simulink model "linear_sim"  (R2024b)
settings: Solver=VariableStepAuto  StartTime=0.0  StopTime=10.0  MaxStep=1e-4  RelTol=1e-3
values from neighbouring files (symbols this model uses):
  c_l_d = 1.5    [linear_params.m]
  K = -lqr(sys,Q,R,0)    [linear_model.m]
  K_pre = 1/dcgain(sys_cl(1,1))    [linear_model.m]
  ref_area = 0.005    [linear_params.m]
  ref_length = 0.25    [linear_params.m]
  rho = 1.293    [linear_params.m]
  tau = 1/60    (= 0.0166666666667)    [linear_params.m]
  V = 100    [linear_model.m]    (also in linear_params.m = 1000)
undefined symbols (not defined in the file or in its folder): backlash, gaussian
libraries: simulink x4, aerolibactuator x1
settings Model: Creator=finnb  LastModifiedBy=finnb

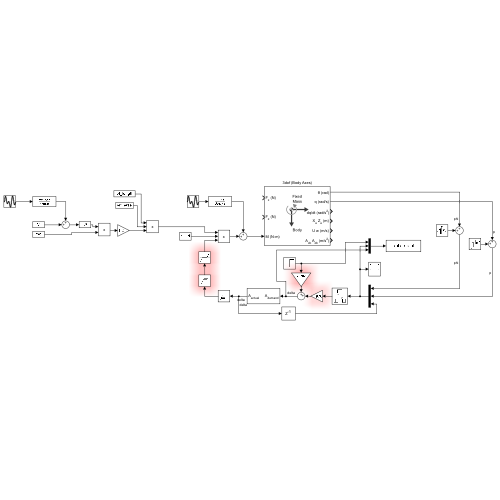
[thumbnail: Simulink's stored preview of the top-level diagram]
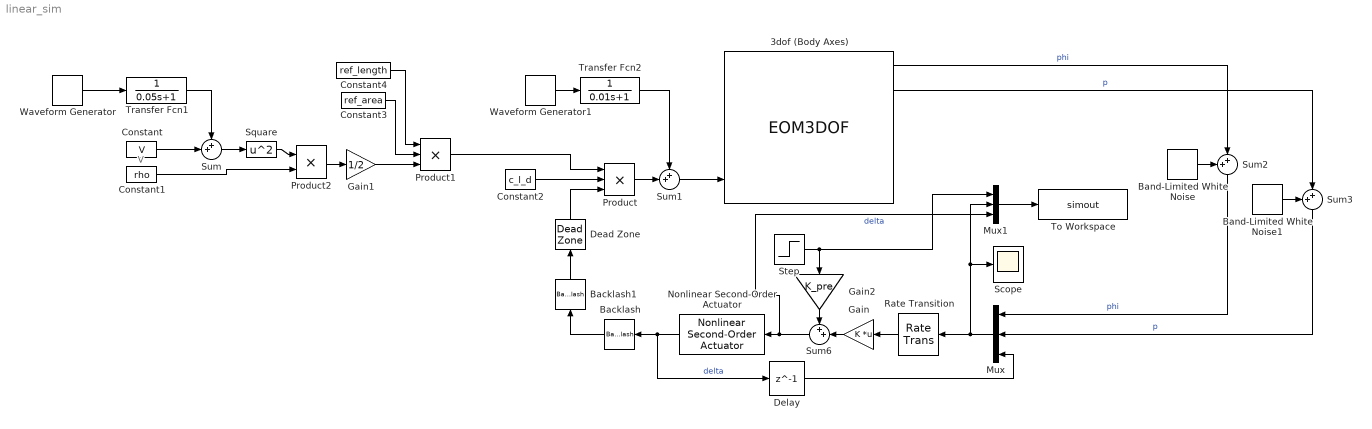
== system linear_sim ==
  note: V
  3dof (Body Axes) : EOM3DOF  v_ini=0  mass=100  Iyy=J  g=0
  Backlash : Backlash  BacklashWidth=pi/180 * 0.5
  Backlash1 : Backlash  BacklashWidth=deg2rad(backlash)
  Band-Limited White Noise : simulink/Sources/Band-Limited White Noise  Cov=[1e-5]  Ts=0.005  seed=[23341]
  Band-Limited White Noise1 : simulink/Sources/Band-Limited White Noise  Cov=[1e-6]  Ts=0.005  seed=[23341]
  Constant : Constant  Value=V
  Constant1 : Constant  Value=rho
  Constant2 : Constant  Value=c_l_d
  Constant3 : Constant  Value=ref_area
  Constant4 : Constant  Value=ref_length
  Dead Zone : DeadZone  LowerValue=-deg2rad(backlash)  UpperValue=deg2rad(backlash)
  Delay : Delay  DelayLength=1  SampleTime=0.005
  Gain : Gain  Gain=K  Multiplication=Matrix(K*u)
  Gain1 : Gain  Gain=1/2
  Gain2 : Gain  Gain=K_pre
  Mux : Mux  Inputs=3
  Mux1 : Mux  Inputs=3
  Nonlinear Second-Order Actuator : aerolibactuator/Nonlinear Second-Order Actuator  wn_fin=1/tau  z_fin=0.9  fin_max=15*pi/180  fin_min=-15*pi/180  fin_maxrate=60/0.1*pi/180  fin_act_0=0  fin_act_vel=0
  Product : Product  Inputs=3
  Product1 : Product  Inputs=3
  Product2 : Product
  Rate Transition : RateTransition  OutPortSampleTime=0.005
  Scope : Scope
  Square : Math  Operator=square
  Step : Step  SampleTime=0
  Sum{,1..3,6} (5 alike) : Sum  Inputs=++|
  To Workspace : ToWorkspace  VariableName=simout  SampleTime=-1
  Transfer Fcn1 : TransferFcn  Denominator=[0.05 1]
  Transfer Fcn2 : TransferFcn  Denominator=[0.01 1]
  Waveform Generator : simulink/Sources/Waveform Generator  OutMin=[]  OutMax=[]  OutDataTypeStr=double  SelectedSignal=1  Signals=gaussian(20,10,1)*2  BlockNames=MultiportSwitch_9246ce97e94b4c1  SampleTime=0.1
  Waveform Generator1 : simulink/Sources/Waveform Generator  OutMin=[]  OutMax=[]  OutDataTypeStr=double  SelectedSignal=1  Signals=gaussian(0.03,0.001,1342)  BlockNames=MultiportSwitch_92ef1fa4760e409  SampleTime=0.1
  wires:
  Mux/1 -> Mux1/2, Scope/1, Rate Transition/1
  Gain/1 -> Sum6/2
  3dof (Body Axes)/1 -> Sum2/2  "phi"
  3dof (Body Axes)/2 -> Sum3/2  "p"
  Constant/1 -> Sum/2
  Constant1/1 -> Product2/2
  Product/1 -> Sum1/2
  Constant2/1 -> Product/2
  Product1/1 -> Product/1
  Product2/1 -> Gain1/1
  Constant3/1 -> Product1/2
  Constant4/1 -> Product1/1
  Waveform Generator/1 -> Transfer Fcn1/1
  Sum/1 -> Square/1
  Sum1/1 -> 3dof (Body Axes)/3
  Waveform Generator1/1 -> Transfer Fcn2/1
  Square/1 -> Product2/1
  Gain1/1 -> Product1/3
  Sum2/1 -> Mux/1  "phi"
  Band-Limited White Noise/1 -> Sum2/1
  Band-Limited White Noise1/1 -> Sum3/1
  Sum3/1 -> Mux/2  "p"
  Gain2/1 -> Sum6/1
  Step/1 -> Mux1/1, Gain2/1
  Rate Transition/1 -> Gain/1
  Nonlinear Second-Order Actuator/1 -> Delay/1, Backlash/1  "delta"
  Sum6/1 -> Mux1/3, Nonlinear Second-Order Actuator/1  "delta"
  Delay/1 -> Mux/3
  Transfer Fcn1/1 -> Sum/1
  Transfer Fcn2/1 -> Sum1/1
  Backlash/1 -> Backlash1/1
  Mux1/1 -> To Workspace/1
  Backlash1/1 -> Dead Zone/1
  Dead Zone/1 -> Product/3
